simulink model "Power_MIL"  (R2024b)
settings: Solver=FixedStepAuto  StartTime=0.0  StopTime=50.0  FixedStep=0.01  RelTol=1e-3
undefined symbols (not defined in the file or in its folder): dcVoltage, Np, Ns, RegulatorLogicControl_12, RegulatorLogicControl_3, RegulatorLogicControl_5, sensor
libraries: nesl_utility x24, fl_lib x21, ee_lib x5, batt_lib x1, autolibdatasheetbattery x1, autolibdcdc x1
(part 1 of 2)
settings Model: Creator=User  LastModifiedBy=User

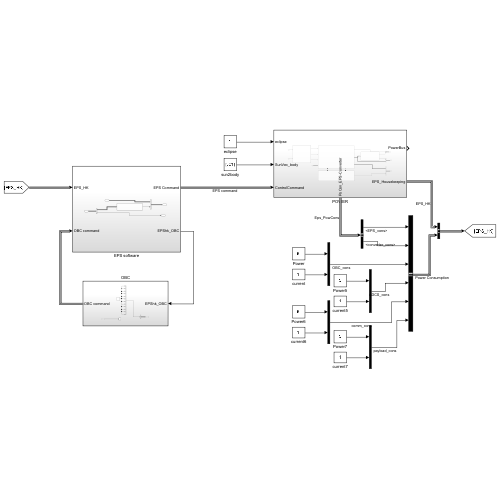
[thumbnail: Simulink's stored preview of the top-level diagram]
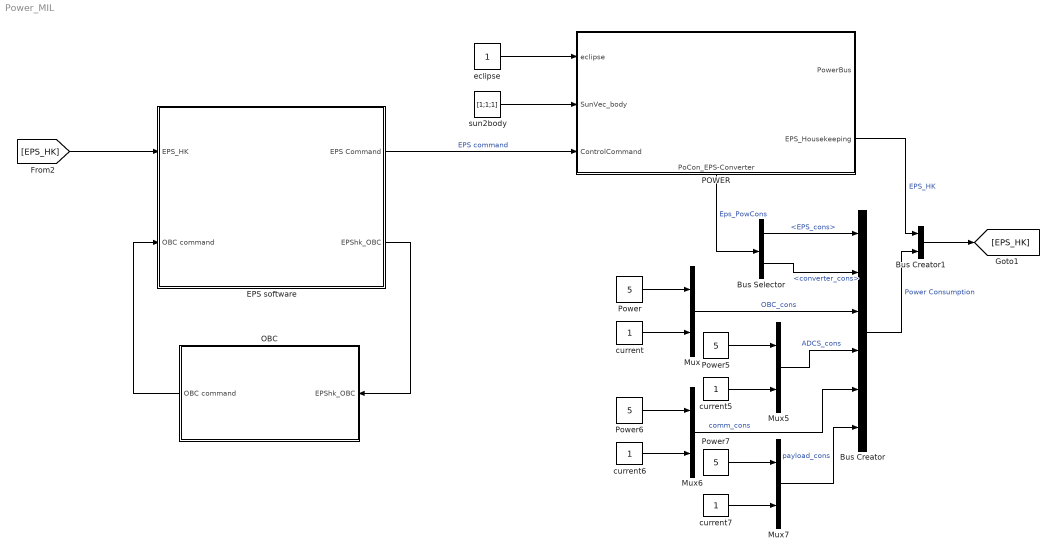
== system Power_MIL ==
  Bus Creator : BusCreator  Inputs=6
  Bus Creator1 : BusCreator  Inputs=2
  Bus Selector : BusSelector  OutputSignals=EPS_cons,converter_cons
  EPS software : Subsystem
  Mux{,5..7} (4 alike) : Mux  Inputs=2
  OBC : Subsystem
  POWER : Subsystem
      settings: PortSchema="{\"entries\":[{\"content\":{\"sides\":[{\"content\":{\"connectorIds\":[\"In1\",\"In2\",\"In3\"]},\"type\":\"ConnectorPlacement.EquallySpacedRectSide\",\"uuid\":\"55b1ea36-8eab-4bc5-8517-9ae39e565ddc\"},{\"content\":{\"connectorIds\":[\"Out1\",\"Out2\"],\"side\":\"RIGHT\"},\"type\":\"ConnectorPlacement.EquallySpacedRectSide\",\"uuid\":\"9643433e-e803-4b91-852a-755e0f780005\"},{\"content\":{\"side\":\"TOP\"},\"type\":\"ConnectorPlacement.EquallySpacedRectSide\",\"uuid\":\"c78c160f-a66a-4ac3-8386-93dfca1751b0\"},{\"content\":{\"connectorIds\":[\"Out3\"],\"side\":\"BOTTOM\"},\"type\":\"ConnectorPlacement.EquallySpacedRectSide\",\"uuid\":\"351da84f-fe2b-4525-9d32-1f07f7d68bc1\"}]},\"type\":\"ConnectorPlacement.EquallySpacedConnector\",\"uuid\":\"3decd512-0aa4-4bce-b130-9054775b0464\"}],\"packageUris\":[\"http://schema.mathworks.com/mf0/Connector/R2020b\"],\"version\":\"1.0\"}"
  Power{,5..7} (4 alike) : Constant  Value=5
  current{,5..7} (4 alike) : Constant
  eclipse : Constant
  sun2body : Constant  Value=[1;1;1]
  wires:
  Bus Creator1/1 -> [EPS_HK]
  EPS software/1(EPS Command) -> POWER/3(ControlCommand)  "EPS command"
  [EPS_HK] -> EPS software/1(EPS_HK)
  EPS software/2(EPShk_OBC) -> OBC/1(EPShk_OBC)
  OBC/1(OBC command) -> EPS software/2(OBC command)
  Power/1 -> Mux/1
  current/1 -> Mux/2
  eclipse/1 -> POWER/1(eclipse)
  sun2body/1 -> POWER/2(SunVec_body)
  Bus Selector/1 -> Bus Creator/1  "<EPS_cons>"
  Bus Selector/2 -> Bus Creator/2  "<converter_cons>"
  current5/1 -> Mux5/2
  Power5/1 -> Mux5/1
  Power6/1 -> Mux6/1
  current6/1 -> Mux6/2
  current7/1 -> Mux7/2
  Power7/1 -> Mux7/1
  Mux/1 -> Bus Creator/3  "OBC_cons"
  Mux5/1 -> Bus Creator/4  "ADCS_cons"
  Mux6/1 -> Bus Creator/5  "comm_cons"
  Mux7/1 -> Bus Creator/6  "payload_cons"
  POWER/2(EPS_Housekeeping) -> Bus Creator1/1  "EPS_HK"
  Bus Creator/1 -> Bus Creator1/2  "Power Consumption"
  POWER/3(PoCon_EPS-Converter) -> Bus Selector/1  "Eps_PowCons"

== system Power_MIL/EPS software ==
  EPS_HK : Inport
  OBC command : Inport  Port=2
  Bus Creator : BusCreator  Inputs=2
  Bus Selector : BusSelector  OutputSignals=Power Consumption,EPS_HK.BatterySOC
  MATLAB Function1 : MATLAB Function  TreatAsAtomicUnit=on
  EPS Command : Outport
  EPShk_OBC : Outport  Port=2
  wires:
  EPS_HK/1 -> Bus Selector/1  "EpsHK"
  Bus Creator/1 -> EPS Command/1
  OBC command/1 -> Bus Creator/1  "OBC_comm"
  MATLAB Function1/1(TotalCurrent) -> Bus Creator/2  "ToT_current"
  Bus Selector/1 -> MATLAB Function1/1(Power_consumption)  "<Power Consumption>"
  Bus Selector/2 -> EPShk_OBC/1  "<BatterySOC>"

== system Power_MIL/OBC ==
  EPShk_OBC : Inport
  Bus Creator : BusCreator  Inputs=1
  Constant : Constant
  Mux : Mux  Inputs=12
  Terminator : Terminator
  OBC command : Outport
  wires:
  Constant/1 -> Mux/12, Mux/11, Mux/10, Mux/9, Mux/8, Mux/7, Mux/4, Mux/3, Mux/1, Mux/2, Mux/5, Mux/6
  Bus Creator/1 -> OBC command/1
  Mux/1 -> Bus Creator/1  "switches_condition"
  EPShk_OBC/1 -> Terminator/1  "EPS"

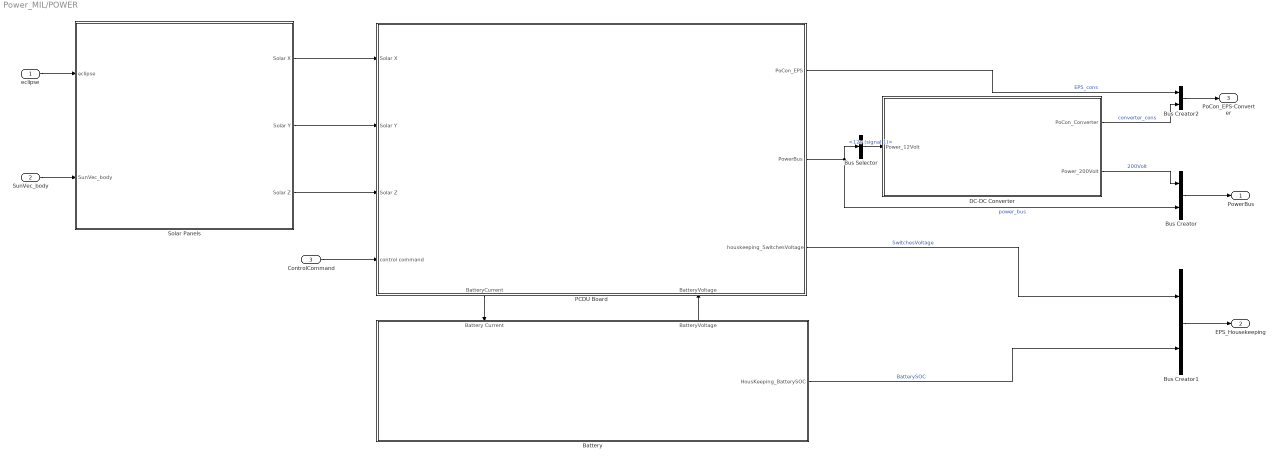
== system Power_MIL/POWER ==
  eclipse : Inport
  SunVec_body : Inport  Port=2
  ControlCommand : Inport  Port=3
  Battery : Subsystem
      settings: PortSchema="{\"entries\":[{\"content\":{\"sides\":[{\"content\":{},\"type\":\"ConnectorPlacement.EquallySpacedRectSide\",\"uuid\":\"aba023eb-c61a-4f67-b0b4-9861c526ec15\"},{\"content\":{\"connectorIds\":[\"Out1\"],\"side\":\"RIGHT\"},\"type\":\"ConnectorPlacement.EquallySpacedRectSide\",\"uuid\":\"3f6535be-9be1-4768-b763-1183b5aa3573\"},{\"content\":{\"connectorIds\":[\"In1\",\"Out2\"],\"side\":\"TOP\"},\"type\":\"ConnectorPlacement.EquallySpacedRectSide\",\"uuid\":\"4513aba4-b806-45fb-9bac-31582bd0c290\"}]},\"type\":\"ConnectorPlacement.EquallySpacedConnector\",\"uuid\":\"e35f9ef2-784c-4297-8a3a-3364ea15e971\"}],\"packageUris\":[\"http://schema.mathworks.com/mf0/Connector/R2020b\"],\"version\":\"1.0\"}"
  Bus Creator : BusCreator  Inputs=2
  Bus Creator1 : BusCreator  Inputs=2
  Bus Creator2 : BusCreator  Inputs=2
  Bus Selector : BusSelector  OutputSignals=12v (signal 1)
  DC-DC Converter : Subsystem
  PCDU Board : Subsystem
      settings: PortSchema="{\"entries\":[{\"content\":{\"sides\":[{\"content\":{\"connectorIds\":[\"In1\",\"In2\",\"In3\",\"In4\"]},\"type\":\"ConnectorPlacement.EquallySpacedRectSide\",\"uuid\":\"36672ca7-eb13-4725-b00c-09a487ba7d91\"},{\"content\":{\"connectorIds\":[\"Out1\",\"Out2\",\"Out3\"],\"side\":\"RIGHT\"},\"type\":\"ConnectorPlacement.EquallySpacedRectSide\",\"uuid\":\"6eafcdb3-9ad1-4020-b7cb-384bf41fe7fc\"},{\"content\":{\"side\":\"TOP\"},\"type\":\"ConnectorPlacement.EquallySpacedRectSide\",\"uuid\":\"e91cfa27-9882-4a24-903a-d0e72077027b\"},{\"content\":{\"connectorIds\":[\"Out4\",\"In5\"],\"side\":\"BOTTOM\"},\"type\":\"ConnectorPlacement.EquallySpacedRectSide\",\"uuid\":\"cff8a778-7a2c-4410-b33c-165bd9362bc6\"}]},\"type\":\"ConnectorPlacement.EquallySpacedConnector\",\"uuid\":\"92ed5259-46ff-4d91-b4a9-1e7fd77d238d\"}],\"packageUris\":[\"http://schema.mathworks.com/mf0/Connector/R2020b\"],\"version\":\"1.0\"}"
  Solar Panels : Subsystem
  PowerBus : Outport
  EPS_Housekeeping : Outport  Port=2
  PoCon_EPS-Converter : Outport  Port=3
  wires:
  eclipse/1 -> Solar Panels/1(eclipse)
  Solar Panels/1(Solar X) -> PCDU Board/1(Solar X)
  Solar Panels/2(Solar Y) -> PCDU Board/2(Solar Y)
  Solar Panels/3(Solar Z) -> PCDU Board/3(Solar Z)
  Bus Creator/1 -> PowerBus/1
  Bus Creator1/1 -> EPS_Housekeeping/1
  ControlCommand/1 -> PCDU Board/4(control command)
  SunVec_body/1 -> Solar Panels/2(SunVec_body)
  Bus Creator2/1 -> PoCon_EPS-Converter/1
  PCDU Board/2(PowerBus) -> Bus Creator/2, Bus Selector/1  "power_bus"
  PCDU Board/4(BatteryCurrent) -> Battery/1(Battery Current)
  Battery/2(BatteryVoltage) -> PCDU Board/5(BatteryVoltage)
  Bus Selector/1 -> DC-DC Converter/1(Power_12Volt)  "<12v (signal 1)>"
  DC-DC Converter/2(Power_200Volt) -> Bus Creator/1  "200Volt"
  PCDU Board/3(houskeeping_SwitchesVoltage) -> Bus Creator1/1  "SwitchesVoltage"
  Battery/1(HousKeeping_BatterySOC) -> Bus Creator1/2  "BatterySOC"
  PCDU Board/1(PoCon_EPS) -> Bus Creator2/1  "EPS_cons"
  DC-DC Converter/1(PoCon_Converter) -> Bus Creator2/2  "converter_cons"

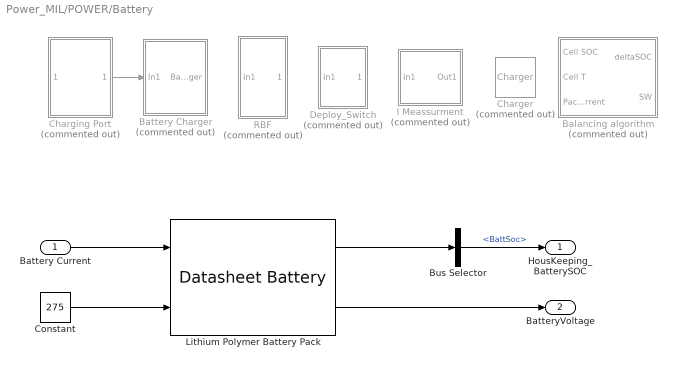
== system Power_MIL/POWER/Battery ==
  Battery Current : Inport
  Balancing algorithm : Subsystem  Commented=on
  Battery Charger : Subsystem  Commented=on
  Bus Selector : BusSelector  OutputSignals=BattSoc
  Charger : batt_lib/Cyclers/Charger  Commented=on  charging_current=5 A  voltage_threshold=12 V  charging_voltage=12 V  current_threshold=0.5 A
      settings: InternalSimscapePortConfiguration="{\"Bottom\":[],\"Left\":[{\"id\":\"trigger\",\"label\":\"t\",\"type\":\"input\"}],\"Right\":[{\"id\":\"p\",\"label\":\"+\",\"type\":\"foundation.electrical.electrical\"},{\"id\":\"n\",\"label\":\"-\",\"type\":\"foundation.electrical.electrical\"}],\"Top\":[]}"
  Charging Port : Subsystem  Commented=on
  Constant : Constant  Value=275
  Deploy_Switch : Subsystem  Commented=on
  I Meassurment : Subsystem  Commented=on
  Lithium Polymer Battery Pack : autolibdatasheetbattery/Datasheet Battery  CapacityCtrl=Parameter  OutputVlt=Unfiltered  BattChargeMax=100  Em=[2.8 3.228 3.284 3.361 3.408 3.427 3.472 3.477 3.493 3.504 3.516 3.528 3.537 3.545 3.555 3.561 3.566 3.576 3.587 3.589 3.594 3.6 3.608 3.61 3.616 3.619 3.626 3.632 3.637 3.64 3.645 3.646 3.652 3.655 3.658 3.661 3.664 3.668 3.673 3.678 3.68 3.681 3.686 3.692 3.699 3.702 3.705 3.71 3.717 3.723 3.728 3.733 3.735 3.742 3.749 3.755 3.761 3.768 3.773 3.78 3.791 3.798 3.798 3.814 3.818 3.825 3.841 3.846 3.855 3.863 3.877 3.885 3.894 3.907 3.919 3.926 3.935 3.944 3.954 3.964 3.974 3.988 3.998 4.014 4.029 4.034 4.047 4.065 4.074 4.086 4.097 4.131 4.126 4.138 4.15 4.18 4.174 4.187 4.207 4.231 4.221]  CapLUTBp=[0 0.01 0.02 0.03 0.04 0.05 0.06 0.07 0.08 0.09 0.1 0.11 0.12 0.13 0.14 0.15 0.16 0.17 0.18 0.19 0.2 0.21 0.22 0.23 0.24 0.25 0.26 0.27 0.28 0.29 0.3 0.31 0.32 0.33 0.34 0.35 0.36 0.37 0.38 0.39 0.4 0.41 0.42 0.43 0.44 0.45 0.46 0.47 0.48 0.49 0.5 0.51 0.52 0.53 0.54 0.55 0.56 0.57 0.58 0.59 0.6 0.61 0.62 0.63 0.64 0.65 0.66 0.67 0.68 0.69 0.7 0.71 0.72 0.73 0.74 0.75 0.76 0.77 0.78 0.79 0.8 0.81 0.82 0.83 0.84 0.85 0.86 0.87 0.88 0.89 0.9 0.91 0.92 0.93 0.94 0.95 0.96 0.97 0.98 0.99 1]  RInt=[0.008846 0.009319 0.009027 0.00847 0.01032 0.01314;0.006389 0.006554 0.005553 0.005525 0.006043 0.007805;0.004364 0.004101 0.00406 0.003452 0.003846 0.004517;0.002031 0.002563 0.002532 0.00246 0.002716 0.003047;0.001443 0.001825 0.001795 0.001778 0.001924 0.002234;0.0005603 0.0007192 0.0006887 0.0007557 0.0007355 0.001014;0.001028 0.001338 0.001 0.001536 0.001546 0.002789]  BattTempBp=[243.1 253.1 263.1 273.1 283.1 298.1 313.1]  CapSOCBp=[0 0.2 0.4 0.6 0.8 1]  Ns=1  Np=1  BattCapInit=100  Tc=1/1000  Vinit=4.221  RefBlkName='autolibdatasheetbattery/Datasheet Battery'
  RBF : Subsystem  Commented=on
  HousKeeping_BatterySOC : Outport
  BatteryVoltage : Outport  Port=2
  wires:
  Lithium Polymer Battery Pack/1 -> Bus Selector/1
  Charging Port/1(Battery_Charger) -> Battery Charger/1(In1)
  Battery Current/1 -> Lithium Polymer Battery Pack/1
  Bus Selector/1 -> HousKeeping_BatterySOC/1  "<BattSoc>"
  Constant/1 -> Lithium Polymer Battery Pack/2
  Lithium Polymer Battery Pack/2 -> BatteryVoltage/1

== system Power_MIL/POWER/DC-DC Converter ==
  Power_12Volt : Inport
  Bidirectional DC-DC : autolibdcdc/Bidirectional DC-DC  Commented=on  Tc=1/1000  Vinit=0  Plimit=100000  param_loss=Single efficiency measurement  eff=98  v_loss_bp=[0 200 400 600 800 1000]  i_loss_bp=[0 25 50 75 100]  losses_table=[100 100 100 100 100;100 150 200 250 300;100 200 300 400 500;100 250 400 550 700;100 300 500 700 900;100 350 600 850 1100]  v_eff_bp=[200 400 600 800 1000]  i_eff_bp=[25 50 75 100]  efficiency_table=[96.2 98.1 98.7 99;98.1 99 99.4 99.5;98.7 99.4 99.6 99.7;99 99.5 99.7 99.8;99.2 99.6 99.7 99.8]  x_v_bp=[-1000 -800 -600 -400 -200 200 400 600 800 1000]  x_i_bp=[-100 -75 -50 -25 25 50 75 100]  x_losses_mat=[200.400801603196 225.67703109328 200.803212851408 201.612903225806 199.999999999997 200 225 200;160.320641282556 180.541624874624 201.005025125625 202.020202020203 200 200 180 160;180.541624874624 180.722891566267 181.086519114686 197.568389057748 194.999999999999 179.999999999997 180 180;201.005025125625 181.086519114686 202.020202020203 193.67991845056 190 200 179.999999999997 200;202.020202020203 197.568389057748 193.67991845056 197.505197505197 190 190 194.999999999999 200;200 194.999999999999 190 190 197.505197505197 193.67991845056 197.568389057748 202.020202020203;200 179.999999999997 200 190 193.67991845056 202.020202020203 181.086519114686 201.005025125625;180 180 179.999999999997 194.999999999999 197.568389057748 181.086519114686 180.722891566267 180.541624874624;160 180 200 200 202.020202020203 201.005025125625 180.541624874624 160.320641282556;200 225 200 199.999999999997 201.612903225806 200.803212851408 225.67703109328 200.400801603196]  RefBlkName='autolibdcdc/Bidirectional DC-DC'  CalLossMapData={'BaseCageProjectFileName','';'BaseMbcProjectFileName','';'TaskName','Calibrate Inverter Loss Map';'ChildTasks',{{'DataName','';'TaskName','Import Loss Data'},{'TaskName','Generate Response Models'},{'TaskName','Generate Calibration'},{'TaskName','Update Block Parameters'}}}
  Divide : Product  Inputs=*/
  Gain : Gain  Gain=200/12
  Mux : Mux  Inputs=2
  Product : Product
  R : Constant
  PoCon_Converter : Outport
  Power_200Volt : Outport  Port=2
  wires:
  R/1 -> Divide/2
  Divide/1 -> Mux/2, Product/2  "current"
  Product/1 -> Mux/1
  Power_12Volt/1 -> Gain/1, Divide/1, Product/1  "Voltage"
  Mux/1 -> PoCon_Converter/1
  Gain/1 -> Power_200Volt/1

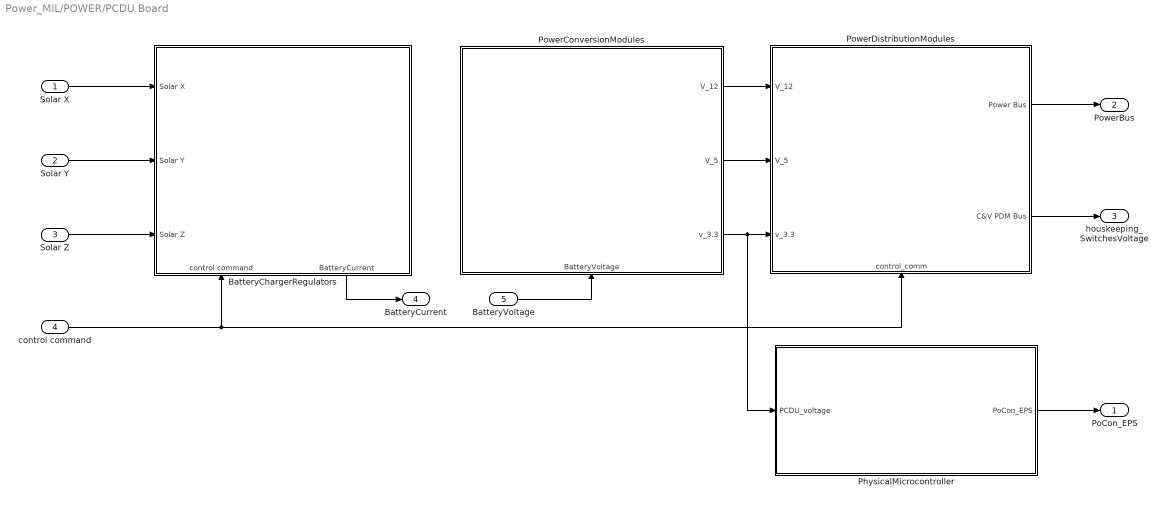
== system Power_MIL/POWER/PCDU Board ==
  Solar X : Inport
  Solar Y : Inport  Port=2
  Solar Z : Inport  Port=3
  control command : Inport  Port=4
  BatteryVoltage : Inport  Port=5
  BatteryChargerRegulators : Subsystem
      settings: PortSchema="{\"entries\":[{\"content\":{\"sides\":[{\"content\":{\"connectorIds\":[\"In1\",\"In2\",\"In3\"]},\"type\":\"ConnectorPlacement.EquallySpacedRectSide\",\"uuid\":\"a54c6477-f532-403d-8d22-fe8c7187031b\"},{\"content\":{\"side\":\"RIGHT\"},\"type\":\"ConnectorPlacement.EquallySpacedRectSide\",\"uuid\":\"77a78f68-d33d-41d0-b8f1-9e3ab7c3612b\"},{\"content\":{\"side\":\"TOP\"},\"type\":\"ConnectorPlacement.EquallySpacedRectSide\",\"uuid\":\"40e6fe94-fdf3-42ac-b4f7-43c530d7ca8e\"},{\"content\":{\"connectorIds\":[\"In4\",\"Out1\"],\"side\":\"BOTTOM\"},\"type\":\"ConnectorPlacement.EquallySpacedRectSide\",\"uuid\":\"5f994662-38e6-4570-aab0-67fb9122f990\"}]},\"type\":\"ConnectorPlacement.EquallySpacedConnector\",\"uuid\":\"6ae65874-5838-4158-9d12-5770a4409470\"}],\"packageUris\":[\"http://schema.mathworks.com/mf0/Connector/R2020b\"],\"version\":\"1.0\"}"
  PhysicalMicrocontroller : Subsystem
  PowerConversionModules : Subsystem
      settings: PortSchema="{\"entries\":[{\"content\":{\"sides\":[{\"content\":{},\"type\":\"ConnectorPlacement.EquallySpacedRectSide\",\"uuid\":\"7faa42b3-e758-4a59-bd59-cf39d4aa9549\"},{\"content\":{\"connectorIds\":[\"Out1\",\"Out2\",\"Out3\"],\"side\":\"RIGHT\"},\"type\":\"ConnectorPlacement.EquallySpacedRectSide\",\"uuid\":\"fd6f184d-0914-459d-a4a5-5106acefe1a2\"},{\"content\":{\"side\":\"TOP\"},\"type\":\"ConnectorPlacement.EquallySpacedRectSide\",\"uuid\":\"8eb7f5a0-03ff-41d6-8f99-6dc2709a1a61\"},{\"content\":{\"connectorIds\":[\"In1\"],\"side\":\"BOTTOM\"},\"type\":\"ConnectorPlacement.EquallySpacedRectSide\",\"uuid\":\"52483d8d-c391-40d7-8f9f-4b93cbeba715\"}]},\"type\":\"ConnectorPlacement.EquallySpacedConnector\",\"uuid\":\"8e205f56-f28b-497f-b412-2c567253f0db\"}],\"packageUris\":[\"http://schema.mathworks.com/mf0/Connector/R2020b\"],\"version\":\"1.0\"}"
  PowerDistributionModules : Subsystem
      settings: PortSchema="{\"entries\":[{\"content\":{\"sides\":[{\"content\":{\"connectorIds\":[\"In1\",\"In2\",\"In3\"]},\"type\":\"ConnectorPlacement.EquallySpacedRectSide\",\"uuid\":\"cc944067-0ae4-44c1-82d9-a1ec81fe8cae\"},{\"content\":{\"connectorIds\":[\"Out1\",\"Out2\"],\"side\":\"RIGHT\"},\"type\":\"ConnectorPlacement.EquallySpacedRectSide\",\"uuid\":\"14a8b3bc-9f23-4806-a571-fc273ce75e66\"},{\"content\":{\"side\":\"TOP\"},\"type\":\"ConnectorPlacement.EquallySpacedRectSide\",\"uuid\":\"d74dfaa3-3ba0-49fd-a7b0-c7f12b34c19f\"},{\"content\":{\"connectorIds\":[\"In4\"],\"side\":\"BOTTOM\"},\"type\":\"ConnectorPlacement.EquallySpacedRectSide\",\"uuid\":\"4657f579-020f-4b4b-b590-abcb58cae511\"}]},\"type\":\"ConnectorPlacement.EquallySpacedConnector\",\"uuid\":\"36922770-3f3d-4d84-84df-ae2b6fb05eab\"}],\"packageUris\":[\"http://schema.mathworks.com/mf0/Connector/R2020b\"],\"version\":\"1.0\"}"
  PoCon_EPS : Outport
  PowerBus : Outport  Port=2
  houskeeping_SwitchesVoltage : Outport  Port=3
  BatteryCurrent : Outport  Port=4
  wires:
  Solar X/1 -> BatteryChargerRegulators/1(Solar X)
  Solar Z/1 -> BatteryChargerRegulators/3(Solar Z)
  PowerDistributionModules/1(Power Bus) -> PowerBus/1
  Solar Y/1 -> BatteryChargerRegulators/2(Solar Y)
  control command/1 -> PowerDistributionModules/4(control_comm), BatteryChargerRegulators/4(control command)
  PowerDistributionModules/2(C&V PDM Bus) -> houskeeping_SwitchesVoltage/1
  PhysicalMicrocontroller/1(PoCon_EPS) -> PoCon_EPS/1
  BatteryChargerRegulators/1(BatteryCurrent) -> BatteryCurrent/1
  PowerConversionModules/3(v_3.3) -> PhysicalMicrocontroller/1(PCDU_voltage), PowerDistributionModules/3(v_3.3)
  BatteryVoltage/1 -> PowerConversionModules/1(BatteryVoltage)
  PowerConversionModules/1(V_12) -> PowerDistributionModules/1(V_12)
  PowerConversionModules/2(V_5) -> PowerDistributionModules/2(V_5)

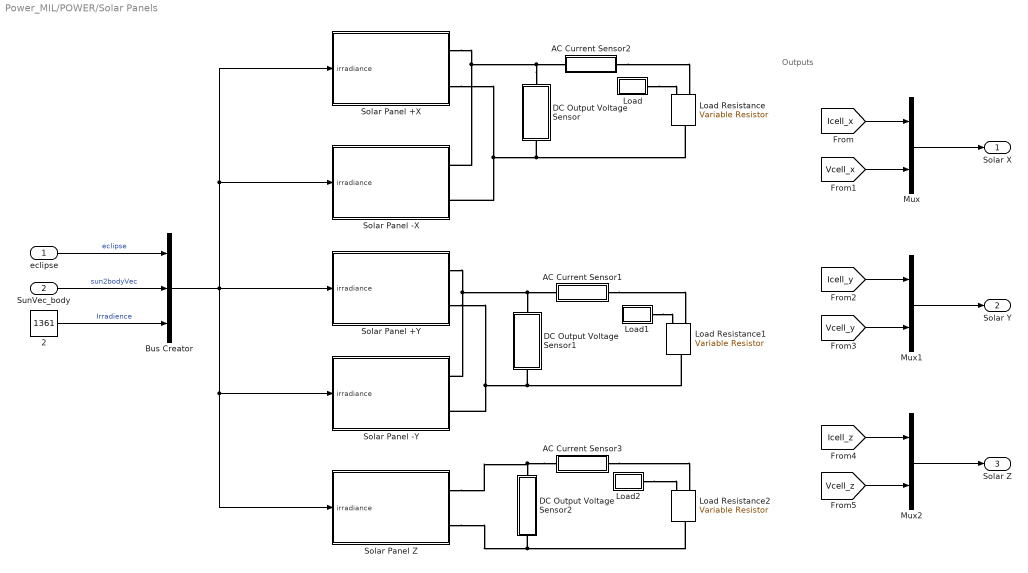
== system Power_MIL/POWER/Solar Panels ==
  note: Outputs
  eclipse : Inport
  SunVec_body : Inport  Port=2
  " 2" : Constant  Value=1361
  AC Current Sensor1 : Subsystem
      mask Display: disp('i');
  AC Current Sensor2 : Subsystem
      mask Display: disp('i');
  AC Current Sensor3 : Subsystem
      mask Display: disp('i');
  Bus Creator : BusCreator  Inputs=3
  DC Output Voltage Sensor : Subsystem
      mask Display: disp('v')
  DC Output Voltage Sensor1 : Subsystem
      mask Display: disp('v')
  DC Output Voltage Sensor2 : Subsystem
      mask Display: disp('v')
  Load : Subsystem
  Load Resistance : fl_lib/Electrical/Electrical Elements/Variable Resistor  Rmin=0 Ohm  thermalEnable=false  thermal_mass=1 J/K  i_specify=off  i_priority=None  i=5 A  i_nominal_specify=off  i_nominal_value=1  i_nominal_unit=A  v_specify=off  v_priority=None  v=0 V  v_nominal_specify=off  v_nominal_value=1  v_nominal_unit=V  T_specify=off  T_priority=None  T=300 K  T_nominal_specify=off  T_nominal_value=1  T_nominal_unit=K
  Load Resistance1 : fl_lib/Electrical/Electrical Elements/Variable Resistor  Rmin=0 Ohm  thermalEnable=false  thermal_mass=1 J/K  i_specify=off  i_priority=None  i=5 A  i_nominal_specify=off  i_nominal_value=1  i_nominal_unit=A  v_specify=off  v_priority=None  v=0 V  v_nominal_specify=off  v_nominal_value=1  v_nominal_unit=V  T_specify=off  T_priority=None  T=300 K  T_nominal_specify=off  T_nominal_value=1  T_nominal_unit=K
  Load Resistance2 : fl_lib/Electrical/Electrical Elements/Variable Resistor  Rmin=0 Ohm  thermalEnable=false  thermal_mass=1 J/K  i_specify=off  i_priority=None  i=5 A  i_nominal_specify=off  i_nominal_value=1  i_nominal_unit=A  v_specify=off  v_priority=None  v=0 V  v_nominal_specify=off  v_nominal_value=1  v_nominal_unit=V  T_specify=off  T_priority=None  T=300 K  T_nominal_specify=off  T_nominal_value=1  T_nominal_unit=K
  Load1 : Subsystem
  Load2 : Subsystem
  Mux : Mux  Inputs=2
  Mux1 : Mux  Inputs=2
  Mux2 : Mux  Inputs=2
  Solar Panel +X : Subsystem
  Solar Panel +Y : Subsystem
  Solar Panel -X : Subsystem
  Solar Panel -Y : Subsystem
  Solar Panel Z : Subsystem
  Solar X : Outport
  Solar Y : Outport  Port=2
  Solar Z : Outport  Port=3
  wires:
  Bus Creator/1 -> Solar Panel -X/1(irradiance), Solar Panel +X/1(irradiance), Solar Panel -Y/1(irradiance), Solar Panel Z/1(irradiance), Solar Panel +Y/1(irradiance)
  [Vcell_y] -> Mux1/2
  [Icell_y] -> Mux1/1
  [Vcell_x] -> Mux/2
  [Icell_x] -> Mux/1
  [Icell_z] -> Mux2/1
  [Vcell_z] -> Mux2/2
  Mux/1 -> Solar X/1
  Mux2/1 -> Solar Z/1
  Mux1/1 -> Solar Y/1
  " 2"/1 -> Bus Creator/3  "Irradience"
  eclipse/1 -> Bus Creator/1  "eclipse"
  SunVec_body/1 -> Bus Creator/2  "sun2bodyVec"
  connections:
  Solar Panel +Y/RConn1 -- Solar Panel -Y/RConn1 -- AC Current Sensor1/RConn1 -- DC Output Voltage Sensor1/RConn1
  DC Output Voltage Sensor/LConn1 -- Solar Panel +X/RConn2 -- Solar Panel -X/RConn2 -- Load Resistance/RConn1
  DC Output Voltage Sensor/RConn1 -- AC Current Sensor2/RConn1 -- Solar Panel +X/RConn1 -- Solar Panel -X/RConn1
  DC Output Voltage Sensor2/LConn1 -- Solar Panel Z/RConn2 -- Load Resistance2/RConn1
  Solar Panel +Y/RConn2 -- Solar Panel -Y/RConn2 -- Load Resistance1/RConn1 -- DC Output Voltage Sensor1/LConn1
  AC Current Sensor3/RConn1 -- Solar Panel Z/RConn1 -- DC Output Voltage Sensor2/RConn1
  AC Current Sensor3/LConn1 -- Load Resistance2/LConn2
  Load/RConn1 -- Load Resistance/LConn1
  AC Current Sensor1/LConn1 -- Load Resistance1/LConn2
  Load2/RConn1 -- Load Resistance2/LConn1
  Load1/RConn1 -- Load Resistance1/LConn1
  AC Current Sensor2/LConn1 -- Load Resistance/LConn2

== system Power_MIL/POWER/Battery/Balancing algorithm ==
  Cell SOC : Inport
  Cell T : Inport  Port=2
  Pack current : Inport  Port=3
  Algorithm : Subsystem
  SOC & T min/max : Subsystem
  deltaSOC : Outport
  SW : Outport  Port=2
  wires:
  Cell SOC/1 -> SOC & T min/max/1(cell SOC)
  Cell T/1 -> SOC & T min/max/2(cell T)
  Pack current/1 -> Algorithm/1(I)
  Algorithm/1(deltaSOC) -> deltaSOC/1
  Algorithm/2(SW) -> SW/1
  SOC & T min/max/1(outBus) -> Algorithm/2(outBus)

== system Power_MIL/POWER/Battery/Battery Charger ==
  In1 : Inport
  Battery_Charger : Outport
  wires:
  In1/1 -> Battery_Charger/1

== system Power_MIL/POWER/Battery/Charging Port ==
  Solar_voltage : Inport
  Battery_Charger : Outport
  wires:
  Solar_voltage/1 -> Battery_Charger/1

== system Power_MIL/POWER/Battery/Deploy_Switch ==
  In1 : Inport
  Out1 : Outport
  wires:
  In1/1 -> Out1/1

== system Power_MIL/POWER/Battery/I Meassurment ==
  In1 : Inport
  Out1 : Outport
  wires:
  In1/1 -> Out1/1

== system Power_MIL/POWER/Battery/RBF ==
  In1 : Inport
  Out1 : Outport
  wires:
  In1/1 -> Out1/1

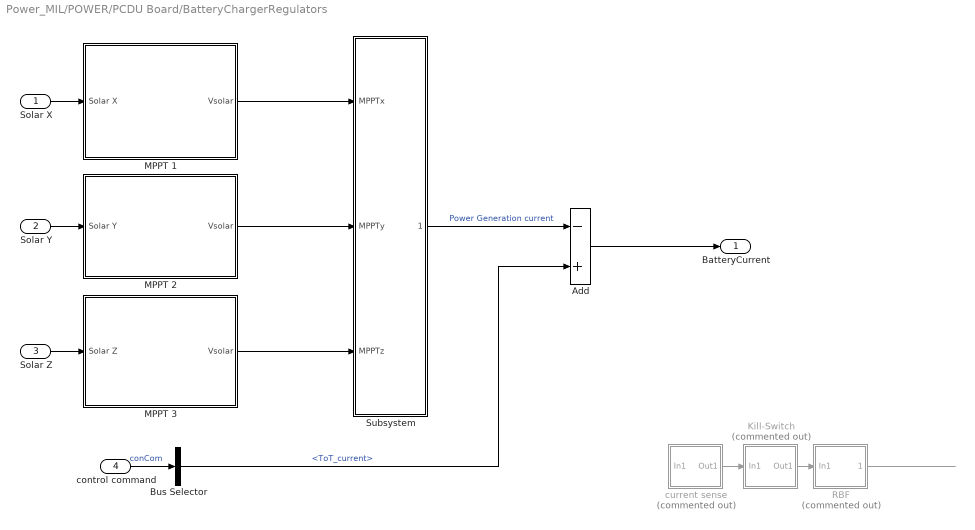
== system Power_MIL/POWER/PCDU Board/BatteryChargerRegulators ==
  Solar X : Inport
  Solar Y : Inport  Port=2
  Solar Z : Inport  Port=3
  control command : Inport  Port=4
  Add : Sum  Inputs=-+
  Bus Selector : BusSelector  OutputSignals=ToT_current
  Kill-Switch : Subsystem  Commented=on
  MPPT 1 : Subsystem
  MPPT 2 : Subsystem
  MPPT 3 : Subsystem
  RBF : Subsystem  Commented=on
  Subsystem : Subsystem
  current sense : Subsystem  Commented=on
  BatteryCurrent : Outport
  wires:
  MPPT 2/1(Vsolar) -> Subsystem/2(MPPTy)
  current sense/1(Out1) -> Kill-Switch/1(In1)
  Add/1 -> BatteryCurrent/1
  MPPT 1/1(Vsolar) -> Subsystem/1(MPPTx)
  Solar Y/1 -> MPPT 2/1(Solar Y)
  RBF/1(Hous Keeping1) -> ?
  Subsystem/1(Solar current) -> Add/1  "Power Generation current"
  Kill-Switch/1(Out1) -> RBF/1(In1)
  MPPT 3/1(Vsolar) -> Subsystem/3(MPPTz)
  Solar X/1 -> MPPT 1/1(Solar X)
  Solar Z/1 -> MPPT 3/1(Solar Z)
  Bus Selector/1 -> Add/2  "<ToT_current>"
  control command/1 -> Bus Selector/1  "conCom"

== system Power_MIL/POWER/PCDU Board/PhysicalMicrocontroller ==
  PCDU_voltage : Inport
  Divide : Product  Inputs=*/
  Mux : Mux  Inputs=2
  Product : Product
  R : Constant
  PoCon_EPS : Outport
  wires:
  PCDU_voltage/1 -> Divide/1, Product/1  "Voltage"
  R/1 -> Divide/2
  Divide/1 -> Mux/2, Product/2  "current"
  Product/1 -> Mux/1  "Power"
  Mux/1 -> PoCon_EPS/1

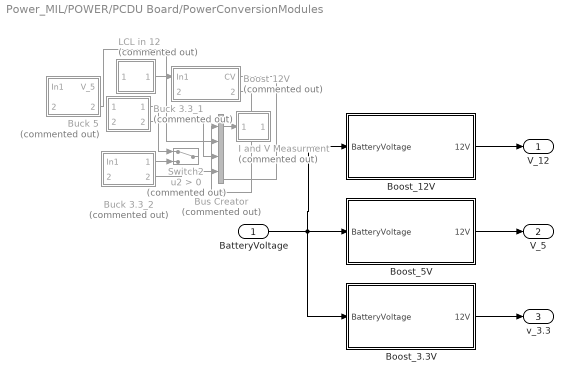
== system Power_MIL/POWER/PCDU Board/PowerConversionModules ==
  BatteryVoltage : Inport
  Boost 12V : Subsystem  Commented=on
  Boost_12V : Subsystem
  Boost_3.3V : Subsystem
  Boost_5V : Subsystem
  Buck 3.3_1 : Subsystem  Commented=on
  Buck 3.3_2 : Subsystem  Commented=on
  Buck 5 : Subsystem  Commented=on
  Bus Creator : BusCreator  Commented=on  Inputs=RegulatorLogicControl_12,RegulatorLogicControl_5,RegulatorLogicControl_3.3_1,RegulatorLogicControl_3.3_2
  I and V Measurment : Subsystem  Commented=on
  LCL in 12 : Subsystem  Commented=on
  Switch2 : Switch  Commented=on  Criteria=u2 > Threshold  SaturateOnIntegerOverflow=off  InputSameDT=off
  V_12 : Outport
  V_5 : Outport  Port=2
  v_3.3 : Outport  Port=3
  wires:
  Buck 3.3_1/1(v_3.3_1) -> Switch2/1
  LCL in 12/1(Out1) -> Boost 12V/1(In1)
  Boost 12V/1(CV) -> I and V Measurment/1(In1)
  Buck 3.3_2/1(Output) -> Switch2/3
  Buck 3.3_1/2(LogicControl_Out) -> Bus Creator/3
  Buck 3.3_2/2(LogicControl_Out) -> Bus Creator/4
  Boost 12V/2(LogicControl_Out) -> Bus Creator/1
  Buck 5/2(LogicControl_Out) -> Bus Creator/2
  BatteryVoltage/1 -> Boost_12V/1(BatteryVoltage), Boost_3.3V/1(BatteryVoltage), Boost_5V/1(BatteryVoltage)
  Boost_12V/1(12V) -> V_12/1
  Boost_5V/1(12V) -> V_5/1
  Boost_3.3V/1(12V) -> v_3.3/1

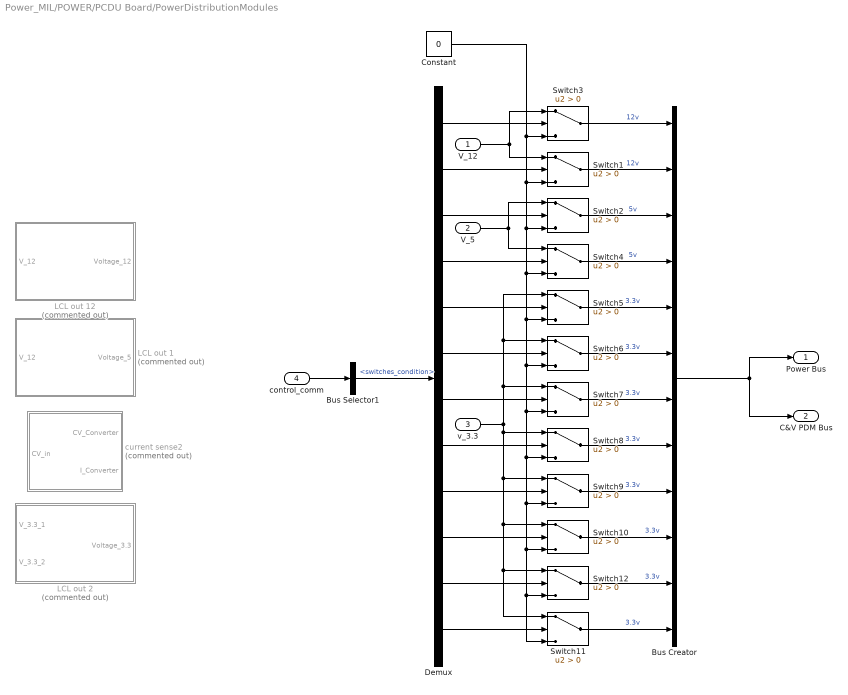
== system Power_MIL/POWER/PCDU Board/PowerDistributionModules ==
  V_12 : Inport
  V_5 : Inport  Port=2
  v_3.3 : Inport  Port=3
  control_comm : Inport  Port=4
  Bus Creator : BusCreator  Inputs=12
  Bus Selector1 : BusSelector  OutputSignals=OBC_comm.switches_condition
  Constant : Constant  Value=0
  Demux : Demux  Outputs=12
  LCL out 1 : Subsystem  Commented=on
  LCL out 12 : Subsystem  Commented=on
  LCL out 2 : Subsystem  Commented=on
  Switch{1..12} (12 alike) : Switch  Criteria=u2 > Threshold  SaturateOnIntegerOverflow=off  InputSameDT=off
  current sense2 : Subsystem  Commented=on
  Power Bus : Outport
  C&V PDM Bus : Outport  Port=2
  wires:
  Bus Creator/1 -> Power Bus/1, C&V PDM Bus/1
  Constant/1 -> Switch11/3, Switch12/3, Switch10/3, Switch9/3, Switch8/3, Switch7/3, Switch6/3, Switch5/3, Switch4/3, Switch2/3, Switch1/3, Switch3/3
  control_comm/1 -> Bus Selector1/1
  Bus Selector1/1 -> Demux/1  "<switches_condition>"
  V_12/1 -> Switch1/1, Switch3/1
  Demux/1 -> Switch3/2
  Demux/2 -> Switch1/2
  V_5/1 -> Switch4/1, Switch2/1
  Demux/3 -> Switch2/2
  v_3.3/1 -> Switch7/1, Switch6/1, Switch5/1, Switch11/1, Switch12/1, Switch10/1, Switch9/1, Switch8/1
  Demux/4 -> Switch4/2
  Demux/5 -> Switch5/2
  Demux/6 -> Switch6/2
  Demux/7 -> Switch7/2
  Demux/8 -> Switch8/2
  Demux/9 -> Switch9/2
  Demux/10 -> Switch10/2
  Demux/11 -> Switch12/2
  Demux/12 -> Switch11/2
  Switch3/1 -> Bus Creator/1  "12v"
  Switch1/1 -> Bus Creator/2  "12v"
  Switch2/1 -> Bus Creator/3  "5v"
  Switch4/1 -> Bus Creator/4  "5v"
  Switch5/1 -> Bus Creator/5  "3.3v"
  Switch6/1 -> Bus Creator/6  "3.3v"
  Switch7/1 -> Bus Creator/7  "3.3v"
  Switch8/1 -> Bus Creator/8  "3.3v"
  Switch9/1 -> Bus Creator/9  "3.3v"
  Switch10/1 -> Bus Creator/10  "3.3v"
  Switch12/1 -> Bus Creator/11  "3.3v"
  Switch11/1 -> Bus Creator/12  "3.3v"

== system Power_MIL/POWER/Solar Panels/AC Current Sensor1 ==
  Current Sensor : fl_lib/Electrical/Electrical Sensors/Current Sensor
  PS-Simulink Converter : nesl_utility/PS-Simulink Converter  PhysicalDomain=network_engine_domain  SubClassName=ps_output  LeftPortType=input  RightPortType=output  PseudoPeriodic=off  Frequencies=[]  VectorFormat=1-D array  Unit=1  AffineConversion=off
  Sensor dynamics : TransferFcn  Numerator=1  Denominator=[1 1]
  - : PMIOPort  Side=Left
  + : PMIOPort  Port=2  Side=Right
  tag scope: Icell_y=global
  wires:
  Sensor dynamics/1 -> [Icell_y]
  PS-Simulink Converter/1 -> Sensor dynamics/1
  connections:
  Current Sensor/RConn2 -- -/RConn1
  +/RConn1 -- Current Sensor/LConn1
  Current Sensor/RConn1 -- PS-Simulink Converter/LConn1

== system Power_MIL/POWER/Solar Panels/AC Current Sensor2 ==
  Current Sensor : fl_lib/Electrical/Electrical Sensors/Current Sensor
  PS-Simulink Converter : nesl_utility/PS-Simulink Converter  PhysicalDomain=network_engine_domain  SubClassName=ps_output  LeftPortType=input  RightPortType=output  PseudoPeriodic=off  Frequencies=[]  VectorFormat=1-D array  Unit=1  AffineConversion=off
  Sensor dynamics : TransferFcn  Numerator=1  Denominator=[1 1]
  Solver Configuration : nesl_utility/Solver Configuration  PhysicalDomain=network_engine_domain  SubClassName=solver  LeftPortType=input  RightPortType=generic  Tones=[]  Harmonics=[]  SimulateNoise=off  Profile=off  UseLocalSampling=off  EnableSwitchedLinearOptims=on  FrequencyDomain=off  UseCCode=off  RelTol=0.001  AbsTol=0.001  MinStep=1e-09  ToWorkspace=off  RevertToSquareIcSolve=off  NumHomotopyIterations=100  PhasorMode=off  PhasorModeNumHarmonics=1  ConsistencySolver=NEWTON_XTOL_AFTER_FTOL  IndexReductionMethod=DerivativeReplacement  DoDC=off  ResidualTolerance=1e-09  ConsistencyTolSource=GLOBAL  ConsistencyAbsTol=0.001  ConsistencyRelTol=0.001  ConsistencyTolFactor=0.001  UseLocalSolver=off  LocalSolverChoice=NE_BACKWARD_EULER_ADVANCER  ResolveIndetEquations=on  FunctionEvalNumThread=1  LocalSolverSampleTime=0.001  DoFixedCost=off  MaxNonlinIter=3  MaxModeIter=2  ComputeImpulses=off  ImpulseIterations=2  LinearAlgebra=auto  LinearAlgebraNumThread=0  EquationFormulation=NE_TIME_EF  DelaysMemoryBudget=1024  AutomaticFiltering=on  FilteringTimeConstant=0.001  PartitionStorageMethod=AS_NEEDED  PartitionMemoryBudget=1024  PartitionMethod=ROBUST  MultibodyUseLocalSolver=off  MultibodyLocalSolverChoice=ODE1  MultibodyLocalSolverSampleTime=0.001
  - : PMIOPort  Side=Left
  + : PMIOPort  Port=2  Side=Right
  tag scope: Icell_x=global
  wires:
  PS-Simulink Converter/1 -> Sensor dynamics/1
  Sensor dynamics/1 -> [Icell_x]
  connections:
  Current Sensor/RConn1 -- Solver Configuration/RConn1 -- PS-Simulink Converter/LConn1
  +/RConn1 -- Current Sensor/LConn1
  Current Sensor/RConn2 -- -/RConn1

== system Power_MIL/POWER/Solar Panels/AC Current Sensor3 ==
  Current Sensor : fl_lib/Electrical/Electrical Sensors/Current Sensor
  PS-Simulink Converter : nesl_utility/PS-Simulink Converter  PhysicalDomain=network_engine_domain  SubClassName=ps_output  LeftPortType=input  RightPortType=output  PseudoPeriodic=off  Frequencies=[]  VectorFormat=1-D array  Unit=1  AffineConversion=off
  Sensor dynamics : TransferFcn  Numerator=1  Denominator=[1 1]
  Solver Configuration : nesl_utility/Solver Configuration  PhysicalDomain=network_engine_domain  SubClassName=solver  LeftPortType=input  RightPortType=generic  Tones=[]  Harmonics=[]  SimulateNoise=off  Profile=off  UseLocalSampling=off  EnableSwitchedLinearOptims=on  FrequencyDomain=off  UseCCode=off  RelTol=0.001  AbsTol=0.001  MinStep=1e-09  ToWorkspace=off  RevertToSquareIcSolve=off  NumHomotopyIterations=100  PhasorMode=off  PhasorModeNumHarmonics=1  ConsistencySolver=NEWTON_XTOL_AFTER_FTOL  IndexReductionMethod=DerivativeReplacement  DoDC=off  ResidualTolerance=1e-09  ConsistencyTolSource=GLOBAL  ConsistencyAbsTol=0.001  ConsistencyRelTol=0.001  ConsistencyTolFactor=0.001  UseLocalSolver=off  LocalSolverChoice=NE_BACKWARD_EULER_ADVANCER  ResolveIndetEquations=on  FunctionEvalNumThread=1  LocalSolverSampleTime=0.001  DoFixedCost=off  MaxNonlinIter=3  MaxModeIter=2  ComputeImpulses=off  ImpulseIterations=2  LinearAlgebra=auto  LinearAlgebraNumThread=0  EquationFormulation=NE_TIME_EF  DelaysMemoryBudget=1024  AutomaticFiltering=on  FilteringTimeConstant=0.001  PartitionStorageMethod=AS_NEEDED  PartitionMemoryBudget=1024  PartitionMethod=ROBUST  MultibodyUseLocalSolver=off  MultibodyLocalSolverChoice=ODE1  MultibodyLocalSolverSampleTime=0.001
  - : PMIOPort  Side=Left
  + : PMIOPort  Port=2  Side=Right
  tag scope: Icell_z=global
  wires:
  PS-Simulink Converter/1 -> Sensor dynamics/1
  Sensor dynamics/1 -> [Icell_z]
  connections:
  Current Sensor/RConn1 -- PS-Simulink Converter/LConn1
  +/RConn1 -- Solver Configuration/RConn1 -- Current Sensor/LConn1
  Current Sensor/RConn2 -- -/RConn1

== system Power_MIL/POWER/Solar Panels/DC Output Voltage Sensor ==
  PS-Simulink Converter : nesl_utility/PS-Simulink Converter  PhysicalDomain=network_engine_domain  SubClassName=ps_output  LeftPortType=input  RightPortType=output  PseudoPeriodic=off  Frequencies=[]  VectorFormat=1-D array  Unit=1  AffineConversion=off
  Sensor dynamics : TransferFcn  Numerator=1  Denominator=[1 1]
  Voltage Sensor : fl_lib/Electrical/Electrical Sensors/Voltage Sensor
  - : PMIOPort  Side=Left
  + : PMIOPort  Port=2  Side=Right
  tag scope: Vcell_x=global
  wires:
  PS-Simulink Converter/1 -> Sensor dynamics/1
  Sensor dynamics/1 -> [Vcell_x]
  connections:
  Voltage Sensor/RConn2 -- -/RConn1
  Voltage Sensor/RConn1 -- PS-Simulink Converter/LConn1
  Voltage Sensor/LConn1 -- +/RConn1

== system Power_MIL/POWER/Solar Panels/DC Output Voltage Sensor1 ==
  PS-Simulink Converter : nesl_utility/PS-Simulink Converter  PhysicalDomain=network_engine_domain  SubClassName=ps_output  LeftPortType=input  RightPortType=output  PseudoPeriodic=off  Frequencies=[]  VectorFormat=1-D array  Unit=1  AffineConversion=off
  Sensor dynamics : TransferFcn  Numerator=1  Denominator=[1 1]
  Voltage Sensor : fl_lib/Electrical/Electrical Sensors/Voltage Sensor
  - : PMIOPort  Side=Left
  + : PMIOPort  Port=2  Side=Right
  tag scope: Vcell_y=global
  wires:
  Sensor dynamics/1 -> [Vcell_y]
  PS-Simulink Converter/1 -> Sensor dynamics/1
  connections:
  Voltage Sensor/LConn1 -- +/RConn1
  Voltage Sensor/RConn1 -- PS-Simulink Converter/LConn1
  Voltage Sensor/RConn2 -- -/RConn1

== system Power_MIL/POWER/Solar Panels/DC Output Voltage Sensor2 ==
  PS-Simulink Converter : nesl_utility/PS-Simulink Converter  PhysicalDomain=network_engine_domain  SubClassName=ps_output  LeftPortType=input  RightPortType=output  PseudoPeriodic=off  Frequencies=[]  VectorFormat=1-D array  Unit=1  AffineConversion=off
  Sensor dynamics : TransferFcn  Numerator=1  Denominator=[1 1]
  Voltage Sensor : fl_lib/Electrical/Electrical Sensors/Voltage Sensor
  - : PMIOPort  Side=Left
  + : PMIOPort  Port=2  Side=Right
  tag scope: Vcell_z=global
  wires:
  PS-Simulink Converter/1 -> Sensor dynamics/1
  Sensor dynamics/1 -> [Vcell_z]
  connections:
  Voltage Sensor/RConn2 -- -/RConn1
  Voltage Sensor/RConn1 -- PS-Simulink Converter/LConn1
  Voltage Sensor/LConn1 -- +/RConn1

== system Power_MIL/POWER/Solar Panels/Load ==
  " " : Constant
  " 1" : Constant  Value=1.5
  Constant : Constant  Value=5
  Load Power (kW) : Gain  Gain=1.688857025146485
  Simulink-PS Converter1 : nesl_utility/Simulink-PS Converter  PhysicalDomain=network_engine_domain  SubClassName=ps_input  LeftPortType=input  RightPortType=output  PseudoPeriodic=off  Frequencies=[]  NoiseDistribution=none  NoiseParameters=[]  Unit=1  AffineConversion=off  FilteringAndDerivatives=provide  SimscapeFilterOrder=1  InputFilterTimeConstant=0.001  UdotUserProvided=0
  Switch : Switch  Criteria=u2 > Threshold  SaturateOnIntegerOverflow=off  InputSameDT=off
  V^2/P : Product  Inputs=*/
  kW2W : Gain  Gain=1000
  R : PMIOPort  Side=Right
  wires:
  " "/1 -> Load Power (kW)/1
  Load Power (kW)/1 -> Switch/1, Switch/2
  " 1"/1 -> Switch/3
  Constant/1 -> V^2/P/1
  V^2/P/1 -> Simulink-PS Converter1/1
  Switch/1 -> kW2W/1
  kW2W/1 -> V^2/P/2
  connections:
  Simulink-PS Converter1/RConn1 -- R/RConn1

== system Power_MIL/POWER/Solar Panels/Load1 ==
  " " : Constant
  " 1" : Constant  Value=1.5
  Constant : Constant  Value=5
  Load Power (kW) : Gain  Gain=1.688857025146485
  Simulink-PS Converter1 : nesl_utility/Simulink-PS Converter  PhysicalDomain=network_engine_domain  SubClassName=ps_input  LeftPortType=input  RightPortType=output  PseudoPeriodic=off  Frequencies=[]  NoiseDistribution=none  NoiseParameters=[]  Unit=1  AffineConversion=off  FilteringAndDerivatives=provide  SimscapeFilterOrder=1  InputFilterTimeConstant=0.001  UdotUserProvided=0
  Switch : Switch  Criteria=u2 > Threshold  SaturateOnIntegerOverflow=off  InputSameDT=off
  V^2/P : Product  Inputs=*/
  kW2W : Gain  Gain=1000
  R : PMIOPort  Side=Right
  wires:
  kW2W/1 -> V^2/P/2
  Switch/1 -> kW2W/1
  V^2/P/1 -> Simulink-PS Converter1/1
  Constant/1 -> V^2/P/1
  " 1"/1 -> Switch/3
  Load Power (kW)/1 -> Switch/2, Switch/1
  " "/1 -> Load Power (kW)/1
  connections:
  Simulink-PS Converter1/RConn1 -- R/RConn1

== system Power_MIL/POWER/Solar Panels/Load2 ==
  " " : Constant
  " 1" : Constant  Value=1.5
  Constant : Constant  Value=5
  Load Power (kW) : Gain  Gain=1.688857025146485
  Simulink-PS Converter1 : nesl_utility/Simulink-PS Converter  PhysicalDomain=network_engine_domain  SubClassName=ps_input  LeftPortType=input  RightPortType=output  PseudoPeriodic=off  Frequencies=[]  NoiseDistribution=none  NoiseParameters=[]  Unit=1  AffineConversion=off  FilteringAndDerivatives=provide  SimscapeFilterOrder=1  InputFilterTimeConstant=0.001  UdotUserProvided=0
  Switch : Switch  Criteria=u2 > Threshold  SaturateOnIntegerOverflow=off  InputSameDT=off
  V^2/P : Product  Inputs=*/
  kW2W : Gain  Gain=1000
  R : PMIOPort  Side=Right
  wires:
  " "/1 -> Load Power (kW)/1
  Load Power (kW)/1 -> Switch/1, Switch/2
  " 1"/1 -> Switch/3
  Constant/1 -> V^2/P/1
  V^2/P/1 -> Simulink-PS Converter1/1
  Switch/1 -> kW2W/1
  kW2W/1 -> V^2/P/2
  connections:
  Simulink-PS Converter1/RConn1 -- R/RConn1

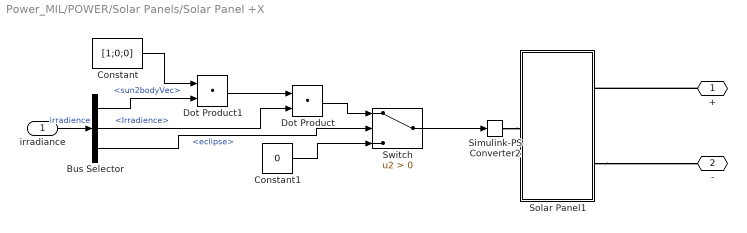
== system Power_MIL/POWER/Solar Panels/Solar Panel +X ==
  irradiance : Inport
  Bus Selector : BusSelector  OutputSignals=sun2bodyVec,Irradience,eclipse
  Constant : Constant  Value=[1;0;0]
  Constant1 : Constant  Value=0
  Dot Product : DotProduct  OutDataTypeStr=Inherit: Inherit via internal rule
  Dot Product1 : DotProduct  OutDataTypeStr=Inherit: Inherit via internal rule
  Simulink-PS Converter2 : nesl_utility/Simulink-PS Converter  PhysicalDomain=network_engine_domain  SubClassName=ps_input  LeftPortType=input  RightPortType=output  PseudoPeriodic=off  Frequencies=[]  NoiseDistribution=none  NoiseParameters=[]  Unit=1  AffineConversion=off  FilteringAndDerivatives=provide  SimscapeFilterOrder=1  InputFilterTimeConstant=0.001  UdotUserProvided=0
  Solar Panel1 : Subsystem  mask(Solar Panel){}
      mask help: Models a solar panel using a parallel-connected string of solar cells. The solar cell strings are modeled using a single Solar Cell block from the Simscape(TM) Electrical(TM) Sources library.
      mask Display: image('ee_solar_panel_icon.jpg')
  Switch : Switch  Criteria=u2 > Threshold  SaturateOnIntegerOverflow=off  InputSameDT=off
  + : PMIOPort  Side=Right
  - : PMIOPort  Port=2  Side=Right
  wires:
  irradiance/1 -> Bus Selector/1  "irradience"
  Dot Product1/1 -> Dot Product/1
  Constant/1 -> Dot Product1/1
  Switch/1 -> Simulink-PS Converter2/1
  Dot Product/1 -> Switch/1
  Constant1/1 -> Switch/3
  Bus Selector/3 -> Switch/2  "<eclipse>"
  Bus Selector/2 -> Dot Product/2  "<Irradience>"
  Bus Selector/1 -> Dot Product1/2  "<sun2bodyVec>"
  connections:
  Simulink-PS Converter2/RConn1 -- Solar Panel1/LConn1
  +/RConn1 -- Solar Panel1/RConn1
  Solar Panel1/RConn2 -- -/RConn1

== system Power_MIL/POWER/Solar Panels/Solar Panel +Y ==
  irradiance : Inport
  Bus Selector1 : BusSelector  OutputSignals=sun2bodyVec,Irradience,eclipse
  Constant : Constant  Value=[0;1;0]
  Constant2 : Constant  Value=0
  Dot Product : DotProduct  OutDataTypeStr=Inherit: Inherit via internal rule
  Dot Product1 : DotProduct  OutDataTypeStr=Inherit: Inherit via internal rule
  Simulink-PS Converter2 : nesl_utility/Simulink-PS Converter  PhysicalDomain=network_engine_domain  SubClassName=ps_input  LeftPortType=input  RightPortType=output  PseudoPeriodic=off  Frequencies=[]  NoiseDistribution=none  NoiseParameters=[]  Unit=1  AffineConversion=off  FilteringAndDerivatives=provide  SimscapeFilterOrder=1  InputFilterTimeConstant=0.001  UdotUserProvided=0
  Solar Panel1 : Subsystem  mask(Solar Panel){}
      mask help: Models a solar panel using a parallel-connected string of solar cells. The solar cell strings are modeled using a single Solar Cell block from the Simscape(TM) Electrical(TM) Sources library.
      mask Display: image('ee_solar_panel_icon.jpg')
  Switch : Switch  Criteria=u2 > Threshold  SaturateOnIntegerOverflow=off  InputSameDT=off
  + : PMIOPort  Side=Right
  - : PMIOPort  Port=2  Side=Right
  wires:
  Bus Selector1/2 -> Dot Product/2  "<Irradience>"
  Bus Selector1/3 -> Switch/2  "<eclipse>"
  Constant/1 -> Dot Product1/1
  Dot Product1/1 -> Dot Product/1
  Switch/1 -> Simulink-PS Converter2/1
  Constant2/1 -> Switch/3
  Dot Product/1 -> Switch/1
  irradiance/1 -> Bus Selector1/1  "irradience"
  Bus Selector1/1 -> Dot Product1/2  "<sun2bodyVec>"
  connections:
  Solar Panel1/LConn1 -- Simulink-PS Converter2/RConn1
  +/RConn1 -- Solar Panel1/RConn1
  Solar Panel1/RConn2 -- -/RConn1

== system Power_MIL/POWER/Solar Panels/Solar Panel -X ==
  irradiance : Inport
  Bus Selector : BusSelector  OutputSignals=sun2bodyVec,Irradience,eclipse
  Constant : Constant  Value=[-1;0;0]
  Constant2 : Constant  Value=0
  Dot Product : DotProduct  OutDataTypeStr=Inherit: Inherit via internal rule
  Dot Product1 : DotProduct  OutDataTypeStr=Inherit: Inherit via internal rule
  Simulink-PS Converter2 : nesl_utility/Simulink-PS Converter  PhysicalDomain=network_engine_domain  SubClassName=ps_input  LeftPortType=input  RightPortType=output  PseudoPeriodic=off  Frequencies=[]  NoiseDistribution=none  NoiseParameters=[]  Unit=1  AffineConversion=off  FilteringAndDerivatives=provide  SimscapeFilterOrder=1  InputFilterTimeConstant=0.001  UdotUserProvided=0
  Solar Panel2 : Subsystem  mask(Solar Panel){}
      mask help: Models a solar panel using a parallel-connected string of solar cells. The solar cell strings are modeled using a single Solar Cell block from the Simscape(TM) Electrical(TM) Sources library.
      mask Display: image('ee_solar_panel_icon.jpg')
  Switch : Switch  Criteria=u2 > Threshold  SaturateOnIntegerOverflow=off  InputSameDT=off
  + : PMIOPort  Side=Right
  - : PMIOPort  Port=2  Side=Right
  wires:
  Bus Selector/2 -> Dot Product/2  "<Irradience>"
  Bus Selector/3 -> Switch/2  "<eclipse>"
  Constant/1 -> Dot Product1/1
  Dot Product1/1 -> Dot Product/1
  Switch/1 -> Simulink-PS Converter2/1
  Constant2/1 -> Switch/3
  Dot Product/1 -> Switch/1
  Bus Selector/1 -> Dot Product1/2  "<sun2bodyVec>"
  irradiance/1 -> Bus Selector/1  "irr"
  connections:
  Solar Panel2/LConn1 -- Simulink-PS Converter2/RConn1
  Solar Panel2/RConn2 -- -/RConn1
  Solar Panel2/RConn1 -- +/RConn1

== system Power_MIL/POWER/Solar Panels/Solar Panel -Y ==
  irradiance : Inport
  Bus Selector : BusSelector  OutputSignals=sun2bodyVec,Irradience,eclipse
  Constant : Constant  Value=[0;-1;0]
  Constant2 : Constant  Value=0
  Dot Product : DotProduct  OutDataTypeStr=Inherit: Inherit via internal rule
  Dot Product1 : DotProduct  OutDataTypeStr=Inherit: Inherit via internal rule
  Simulink-PS Converter2 : nesl_utility/Simulink-PS Converter  PhysicalDomain=network_engine_domain  SubClassName=ps_input  LeftPortType=input  RightPortType=output  PseudoPeriodic=off  Frequencies=[]  NoiseDistribution=none  NoiseParameters=[]  Unit=1  AffineConversion=off  FilteringAndDerivatives=provide  SimscapeFilterOrder=1  InputFilterTimeConstant=0.001  UdotUserProvided=0
  Solar Panel1 : Subsystem  mask(Solar Panel){}
      mask help: Models a solar panel using a parallel-connected string of solar cells. The solar cell strings are modeled using a single Solar Cell block from the Simscape(TM) Electrical(TM) Sources library.
      mask Display: image('ee_solar_panel_icon.jpg')
  Switch : Switch  Criteria=u2 > Threshold  SaturateOnIntegerOverflow=off  InputSameDT=off
  + : PMIOPort  Side=Right
  - : PMIOPort  Port=2  Side=Right
  wires:
  Bus Selector/2 -> Dot Product/2  "<Irradience>"
  Bus Selector/3 -> Switch/2  "<eclipse>"
  Constant/1 -> Dot Product1/1
  Dot Product1/1 -> Dot Product/1
  Switch/1 -> Simulink-PS Converter2/1
  Constant2/1 -> Switch/3
  Dot Product/1 -> Switch/1
  irradiance/1 -> Bus Selector/1  "irradience"
  Bus Selector/1 -> Dot Product1/2  "<sun2bodyVec>"
  connections:
  Solar Panel1/LConn1 -- Simulink-PS Converter2/RConn1
  Solar Panel1/RConn1 -- +/RConn1
  -/RConn1 -- Solar Panel1/RConn2

== system Power_MIL/POWER/Solar Panels/Solar Panel Z ==
  irradiance : Inport
  Bus Selector : BusSelector  OutputSignals=sun2bodyVec,eclipse,Irradience
  Constant : Constant  Value=[0;0;1]
  Constant2 : Constant  Value=0
  Dot Product : DotProduct  OutDataTypeStr=Inherit: Inherit via internal rule
  Dot Product1 : DotProduct  OutDataTypeStr=Inherit: Inherit via internal rule
  Simulink-PS Converter2 : nesl_utility/Simulink-PS Converter  PhysicalDomain=network_engine_domain  SubClassName=ps_input  LeftPortType=input  RightPortType=output  PseudoPeriodic=off  Frequencies=[]  NoiseDistribution=none  NoiseParameters=[]  Unit=1  AffineConversion=off  FilteringAndDerivatives=provide  SimscapeFilterOrder=1  InputFilterTimeConstant=0.001  UdotUserProvided=0
  Solar Panel1 : Subsystem  mask(Solar Panel){}
      mask help: Models a solar panel using a parallel-connected string of solar cells. The solar cell strings are modeled using a single Solar Cell block from the Simscape(TM) Electrical(TM) Sources library.
      mask Display: image('ee_solar_panel_icon.jpg')
  Switch : Switch  Criteria=u2 > Threshold  SaturateOnIntegerOverflow=off  InputSameDT=off
  + : PMIOPort  Side=Right
  - : PMIOPort  Port=2  Side=Right
  wires:
  Bus Selector/3 -> Switch/2  "<Irradience>"
  Constant/1 -> Dot Product1/1
  Dot Product1/1 -> Dot Product/1
  Switch/1 -> Simulink-PS Converter2/1
  Constant2/1 -> Switch/3
  Dot Product/1 -> Switch/1
  irradiance/1 -> Bus Selector/1  "irr"
  Bus Selector/1 -> Dot Product1/2  "<sun2bodyVec>"
  Bus Selector/2 -> Dot Product/2  "<eclipse>"
  connections:
  Solar Panel1/LConn1 -- Simulink-PS Converter2/RConn1
  Solar Panel1/RConn1 -- +/RConn1
  Solar Panel1/RConn2 -- -/RConn1

== system Power_MIL/POWER/Battery/Balancing algorithm/Algorithm ==
  I : Inport
  In Bus Element : Inport  Port=2  PortName=outBus  Element=minSOC
  In Bus Element1 : Inport  Port=2  PortName=outBus  Element=indx_minSOC
  In Bus Element2 : Inport  Port=2  PortName=outBus  Element=maxSOC
  In Bus Element3 : Inport  Port=2  PortName=outBus  Element=indx_maxSOC
  In Bus Element4 : Inport  Port=2  PortName=outBus  Element=minCellT
  In Bus Element5 : Inport  Port=2  PortName=outBus  Element=maxCellT
  Cell Balancing Algorithm : MATLAB Function  TreatAsAtomicUnit=on
  deltaSOC : Outport
  SW : Outport  Port=2
  wires:
  Cell Balancing Algorithm/1(deltaSOC) -> deltaSOC/1
  Cell Balancing Algorithm/2(SW) -> SW/1
  In Bus Element/1 -> Cell Balancing Algorithm/2(minSOC)
  In Bus Element1/1 -> Cell Balancing Algorithm/3(indx_minSOC)
  In Bus Element2/1 -> Cell Balancing Algorithm/4(maxSOC)
  In Bus Element3/1 -> Cell Balancing Algorithm/5(indx_maxSOC)
  In Bus Element4/1 -> Cell Balancing Algorithm/6(minT)
  In Bus Element5/1 -> Cell Balancing Algorithm/7(maxT)
  I/1 -> Cell Balancing Algorithm/1(I)

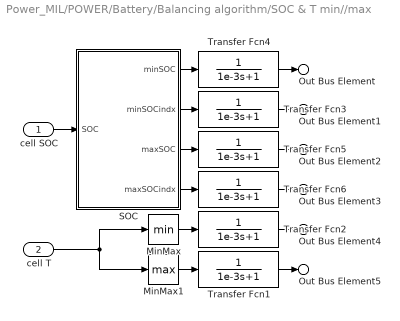
== system Power_MIL/POWER/Battery/Balancing algorithm/SOC & T min//max ==
  cell SOC : Inport
  cell T : Inport  Port=2
  MinMax : MinMax
  MinMax1 : MinMax  Function=max
  SOC : MATLAB Function  TreatAsAtomicUnit=on
  Transfer Fcn{1..6} (6 alike) : TransferFcn  Denominator=[1e-3 1]
  Out Bus Element : Outport  PortName=outBus  Element=minSOC
  Out Bus Element1 : Outport  PortName=outBus  Element=indx_minSOC
  Out Bus Element2 : Outport  PortName=outBus  Element=maxSOC
  Out Bus Element3 : Outport  PortName=outBus  Element=indx_maxSOC
  Out Bus Element5 : Outport  PortName=outBus  Element=minCellT
  Out Bus Element4 : Outport  PortName=outBus  Element=maxCellT
  wires:
  SOC/2(minSOCindx) -> Transfer Fcn3/1
  Transfer Fcn5/1 -> Out Bus Element2/1
  SOC/4(maxSOCindx) -> Transfer Fcn6/1
  SOC/3(maxSOC) -> Transfer Fcn5/1
  cell T/1 -> MinMax/1, MinMax1/1
  Transfer Fcn4/1 -> Out Bus Element/1
  Transfer Fcn3/1 -> Out Bus Element1/1
  SOC/1(minSOC) -> Transfer Fcn4/1
  MinMax/1 -> Transfer Fcn2/1
  MinMax1/1 -> Transfer Fcn1/1
  cell SOC/1 -> SOC/1(SOC)
  Transfer Fcn6/1 -> Out Bus Element3/1
  Transfer Fcn2/1 -> Out Bus Element4/1
  Transfer Fcn1/1 -> Out Bus Element5/1

== system Power_MIL/POWER/PCDU Board/BatteryChargerRegulators/Kill-Switch ==
  In1 : Inport
  Out1 : Outport
  wires:
  In1/1 -> Out1/1
